simulink subsystem "RoboRio_Controls_sub"  (R2023b)
settings: Solver=VariableStepAuto  StartTime=0.0  StopTime=10.0  RelTol=1e-3
undefined symbols (not defined in the file): Odometry_IC_X, Odometry_IC_Y
libraries: simulink x4, Autonomous_lib x1, Disabled_lib x1, Teleop_lib x1, Test_lib x1
(part 1 of 2)
settings Model: Creator=USER  LastModifiedBy=ander

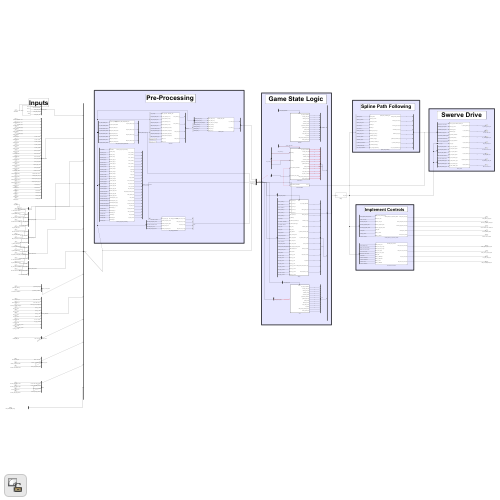
[thumbnail: Simulink's stored preview of the top-level diagram]
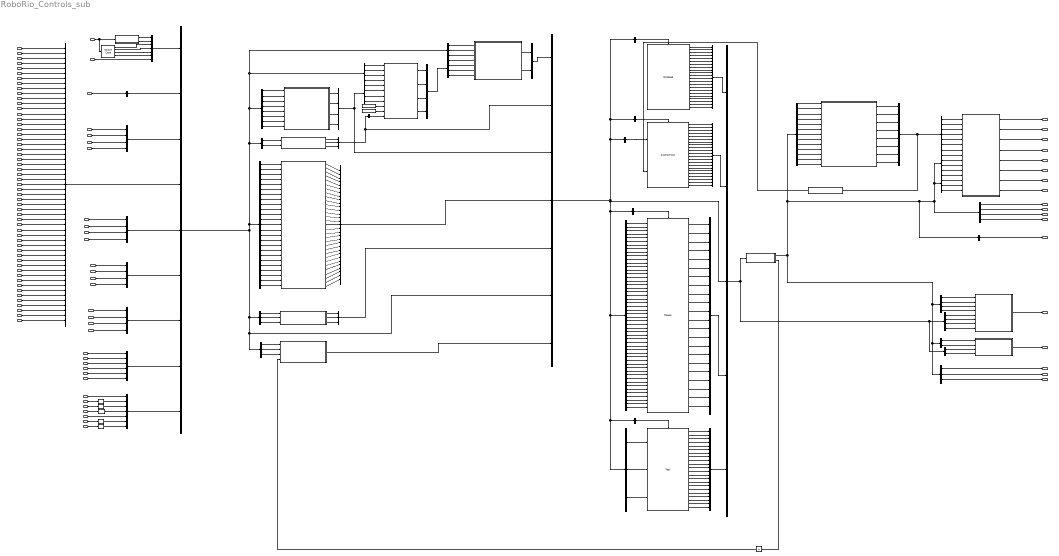
== system RoboRio_Controls_sub ==
  note: Game State Logic
  note: Swerve Drive
  note: Inputs
  note: Pre-Processing
  note: Spline Path
      | Following
  note: Reefscape
  GameState : Inport
  IsBlueAlliance : Inport  Port=2
  Joystick_Left_X : Inport  Port=3
  Joystick_Left_Y : Inport  Port=4
  Joystick_Left_Z : Inport  Port=5
  Joystick_Right_X : Inport  Port=6
  Joystick_Right_Y : Inport  Port=7
  Joystick_Right_Z : Inport  Port=8
  Joystick_Left_B1 : Inport  Port=9
  Joystick_Left_B2 : Inport  Port=10
  Joystick_Left_B3 : Inport  Port=11
  Joystick_Left_B4 : Inport  Port=12
  Joystick_Left_B5 : Inport  Port=13
  Joystick_Left_B6 : Inport  Port=14
  Joystick_Left_B7 : Inport  Port=15
  Joystick_Left_B8 : Inport  Port=16
  Joystick_Left_B9 : Inport  Port=17
  Joystick_Left_B10 : Inport  Port=18
  Joystick_Left_B11 : Inport  Port=19
  Joystick_Left_B12 : Inport  Port=20
  Joystick_Left_B13 : Inport  Port=21
  Joystick_Left_B14 : Inport  Port=22
  Joystick_Left_B15 : Inport  Port=23
  Joystick_Left_B16 : Inport  Port=24
  Joystick_Left_POV : Inport  Port=25
  Joystick_Right_B1 : Inport  Port=26
  Joystick_Right_B2 : Inport  Port=27
  Joystick_Right_B3 : Inport  Port=28
  Joystick_Right_B4 : Inport  Port=29
  Joystick_Right_B5 : Inport  Port=30
  Joystick_Right_B6 : Inport  Port=31
  Joystick_Right_B7 : Inport  Port=32
  Joystick_Right_B8 : Inport  Port=33
  Joystick_Right_B9 : Inport  Port=34
  Joystick_Right_B10 : Inport  Port=35
  Joystick_Right_B11 : Inport  Port=36
  Joystick_Right_B12 : Inport  Port=37
  Joystick_Right_B13 : Inport  Port=38
  Joystick_Right_B14 : Inport  Port=39
  Joystick_Right_B15 : Inport  Port=40
  Joystick_Right_B16 : Inport  Port=41
  Joystick_Right_POV : Inport  Port=42
  Gamepad_Stick_Left_X : Inport  Port=43
  Gamepad_Stick_Left_Y : Inport  Port=44
  Gamepad_Stick_Right_X : Inport  Port=45
  Gamepad_Stick_Right_Y : Inport  Port=46
  Gamepad_B1_A : Inport  Port=47
  Gamepad_B2_B : Inport  Port=48
  Gamepad_B3_X : Inport  Port=49
  Gamepad_B4_Y : Inport  Port=50
  Gamepad_LB : Inport  Port=51
  Gamepad_LT : Inport  Port=52
  Gamepad_RB : Inport  Port=53
  Gamepad_RT : Inport  Port=54
  Gamepad_Back : Inport  Port=55
  Gamepad_Start : Inport  Port=56
  Gamepad_POV : Inport  Port=57
  Gyro_Angle : Inport  Port=58
  FL_Drive_Motor_Speed : Inport  Port=59
  FR_Drive_Motor_Speed : Inport  Port=60
  BL_Drive_Motor_Speed : Inport  Port=61
  BR_Drive_Motor_Speed : Inport  Port=62
  FL_Drive_Motor_Rev : Inport  Port=63
  FR_Drive_Motor_Rev : Inport  Port=64
  BL_Drive_Motor_Rev : Inport  Port=65
  BR_Drive_Motor_Rev : Inport  Port=66
  FL_Steer_Module_Rev : Inport  Port=67
  FR_Steer_Module_Rev : Inport  Port=68
  BL_Steer_Module_Rev : Inport  Port=69
  BR_Steer_Module_Rev : Inport  Port=70
  FL_Steer_Module_Offset : Inport  Port=71
  FR_Steer_Module_Offset : Inport  Port=72
  BL_Steer_Module_Offset : Inport  Port=73
  BR_Steer_Module_Offset : Inport  Port=74
  Limelight_Est_Pose_X : Inport  Port=75
  Limelight_Est_Pose_Y : Inport  Port=76
  Num_Tags_Detected : Inport  Port=77
  Limelight_Tag_X : Inport  Port=78
  Limelight_Tag_Y : Inport  Port=79
  Limelight_Tag_Angle : Inport  Port=80
  Elevator_Motor_Rev : Inport  Port=81
  Elevator_Limit_Switch_Bottom : Inport  Port=82
  Elevator_Limit_Switch_Top : Inport  Port=83
  Coral_Arm_Angle_Measured_Raw : Inport  Port=84
  Coral_TOF_Distance : Inport  Port=85
  Coral_Limit_Switch : Inport  Port=86
  Algae_Limit_Switch : Inport  Port=87
  Add Constant : Bias  Bias=-180  SaturateOnIntegerOverflow=off
  Autonomous : Autonomous_lib/Autonomous  SystemSampleTime=-1  VariantActivationTime=update diagram  AllowFlexibleInterface=on  Latency=0  AutoFrameSizeCalculation=off
  Bus Creator : BusCreator  Inputs=7
  Bus Creator{1..2,4,12} (4 alike) : BusCreator  Inputs=22
  Bus Creator10 : BusCreator  Inputs=7
  Bus Creator11 : BusCreator  Inputs=9
  Bus Creator13 : BusCreator  Inputs=8
  Bus Creator{7..9,14..16} (6 alike) : BusCreator  Inputs=4
  Bus Creator17 : BusCreator  Inputs=7
  Bus Creator18 : BusCreator  Inputs=6
  Bus Creator19 : BusCreator  Inputs=2
  Bus Creator20 : BusCreator  Inputs=3
  Bus Creator21 : BusCreator  Inputs=3
  Bus Creator24 : BusCreator  Inputs=31
  Bus Creator3 : BusCreator  Inputs=5
  Bus Creator5 : BusCreator  Inputs=55
  Bus Creator6 : BusCreator  Inputs=1
  Bus Selector : BusSelector  OutputSignals=Steering_Abs_Cmd_SPF,Steering_Rel_Cmd_SPF,Translation_Speed_SPF,Translation_Angle_SPF,Is_Absolute_Translation_SPF,Is_Absolute_Steering_SPF,Gyro_Angle_SPF
  Bus Selector1 : BusSelector  OutputSignals=Odom_Position_X,Odom_Position_Y,Odom_Delta_X,Odom_Delta_Y
  Bus Selector10 : BusSelector  OutputSignals=Reefscape_Motors_Enable,Elevator_Height_Desired,Coral_Arm_Angle_Desired,Coral_Pickup_Lower_Wait_State
  Bus Selector11 : BusSelector  OutputSignals=Coral_Wheel_DutyCycle,Algae_Wheel_Outside_DutyCycle,Algae_Wheel_Inside_DutyCycle
  Bus Selector12 : BusSelector  OutputSignals=Reefscape_Motors_Enable,Coral_Arm_Angle_Desired
  Bus Selector13 : BusSelector  OutputSignals=Human_Inputs_Raw.Joystick_Left_X,Human_Inputs_Raw.Joystick_Left_Y,Human_Inputs_Raw.Joystick_Left_Z,Human_Inputs_Raw.Joystick_Right_X,Human_Inputs_Raw.Joystick_Right_Y,Human_Inputs_Raw.Joystick_Right_Z,Human_Inputs_Raw.Joystick_Left_B1,Human_Inputs_Raw.Joystick_Left_B2,Human_Inputs_Raw.Joystick_Left_B3,Human_Inputs_Raw.Joystick_Left_B4,Human_Inputs_Raw.Joystick_Left_B11,Human_Inputs_Raw.Joystick_Left_B12,Human_Inputs_Raw.Joystick_Left_B13,Human_Inputs_Raw.Joystick_Left_POV,Human_Inputs_Raw.Joystick_Right_B2,Human_Inputs_Raw.Joystick_Right_B3,Human_Inputs_Raw.Joystick_Right_B4,Human_Inputs_Raw.Joystick_Right_B5,Human_Inputs_Raw.Joystick_Right_B6,Human_Inputs_Raw.Joystick_Right_B7,Human_Inputs_Raw.Joystick_Right_B8,Human_Inputs_Raw.Joystick_Right_B9,Human_Inputs_Raw.Joystick_Right_B10,Human_Inputs_Raw.Joystick_Right_POV,Human_Inputs_Raw.Gamepad_POV
  Bus Selector14 : BusSelector  OutputSignals=PreProcessing.Inputs.Reefscape.Coral_Arm_Angle_Measured,PreProcessing.Elevator_Height_Measured
  Bus Selector15 : BusSelector  OutputSignals=PreProcessing.Gyro.Gyro_Angle_Offset_Total
  Bus Selector16 : BusSelector  OutputSignals=Human_Inputs_Processed.Button_Enable_Wheels,Human_Inputs_Processed.Button_Reset_Wheel_Offsets,Human_Inputs_Processed.Button_Disable_Wheels
  Bus Selector17 : BusSelector  OutputSignals=IMU_Sensor.Gyro_Angle_deg,Game_States.IsBlueAlliance
  Bus Selector18 : BusSelector  OutputSignals=Enable_Wheels,Reset_Wheel_Offsets,Disable_Wheels,Swerve_Motors_Disabled
  Bus Selector19 : BusSelector  OutputSignals=Gyro_Angle_Field_rad
  Bus Selector2 : BusSelector  OutputSignals=Inputs.Game_States.Game_State_Teleop
  Bus Selector20 : BusSelector  OutputSignals=Limelight_Estimates.Limelight_Tag_X,Limelight_Estimates.Limelight_Tag_Y,Limelight_Estimates.Limelight_Tag_Angle
  Bus Selector3 : BusSelector  OutputSignals=Limelight_Estimates.Limelight_Est_Pose_X,Limelight_Estimates.Limelight_Est_Pose_Y,Limelight_Estimates.Num_Tags_Detected
  Bus Selector4 : BusSelector  OutputSignals=Inputs.Game_States.Game_State_Auto
  Bus Selector40 : BusSelector  OutputSignals=Drive_Motor_Revs.FL_Drive_Motor_Rev,Drive_Motor_Revs.FR_Drive_Motor_Rev,Drive_Motor_Revs.BL_Drive_Motor_Rev,Drive_Motor_Revs.BR_Drive_Motor_Rev
  Bus Selector41 : BusSelector  OutputSignals=Human_Inputs_Processed.Drive_Joystick_X,Human_Inputs_Processed.Drive_Joystick_Y,Human_Inputs_Processed.Drive_Joystick_Z,Human_Inputs_Processed.Drive_Joystick_Z_Mode,Human_Inputs_Processed.Steer_Joystick_X,Human_Inputs_Processed.Steer_Joystick_Y,Human_Inputs_Processed.Steer_Joystick_Z,Human_Inputs_Processed.Is_Boosting,Human_Inputs_Processed.Face_Toward_Driver,Human_Inputs_Processed.Face_Right_Driver,Human_Inputs_Processed.Face_Left_Driver,Human_Inputs_Processed.Face_Away_Driver,Gyro.Gyro_Angle_rad,Inputs.Game_States.Prev_GameState,Inputs.Game_States.IsBlueAlliance,EKF.KF_Position_X,EKF.KF_Position_Y,Limelight_Tag_Corrected.Limelight_Tag_Corrected_X,Limelight_Tag_Corrected.Limelight_Tag_Corrected_Y,Limelight_Tag_Corrected.Limelight_Tag_Corrected_Angle,Human_Inputs_Processed.Align_Left,Human_Inputs_Processed.Align_Right,Human_Inputs_Processed.Align_Center,Human_Inputs_Processed.Coral_Station_Left,Human_Inputs_Processed.Coral_Station_Right,Human_Inputs_Processed.Processor,Human_Inputs_Processed.Cage_Left_Start,Human_Inputs_Processed.Cage_Middle_Start,Human_Inputs_Processed.Cage_Right_Start,Human_Inputs_Processed.Cage_Left_Finish,Human_Inputs_Processed.Cage_Middle_Finish,Human_Inputs_Processed.Cage_Right_Finish,Inputs.Human_Inputs_Raw.Gamepad_B1_A,Inputs.Human_Inputs_Raw.Gamepad_B2_B,Inputs.Human_Inputs_Raw.Gamepad_B3_X,Inputs.Human_Inputs_Raw.Gamepad_B4_Y,Inputs.Human_Inputs_Raw.Gamepad_Start,Inputs.Human_Inputs_Raw.Gamepad_Back,Inputs.Human_Inputs_Raw.Gamepad_RB,Inputs.Human_Inputs_Raw.Gamepad_LT,Inputs.Human_Inputs_Raw.Gamepad_RT,Human_Inputs_Processed.Gamepad_POV_Up,Human_Inputs_Processed.Gamepad_POV_Down,Human_Inputs_Processed.Gamepad_POV_Left,Human_Inputs_Processed.Gamepad_POV_Right,Inputs.Human_Inputs_Raw.Gamepad_Stick_Left_Y,Inputs.Human_Inputs_Raw.Gamepad_Stick_Right_Y,Elevator_Height_Measured,Inputs.Reefscape.Coral_Arm_Angle_Measured,Inputs.Reefscape.Coral_TOF_Distance,Inputs.Reefscape.Coral_Limit_Switch,Inputs.Reefscape.Algae_Limit_Switch
  Bus Selector5 : BusSelector  OutputSignals=Reefscape.Elevator_Motor_Rev,Reefscape.Elevator_Limit_Switch_Bottom,Reefscape.Elevator_Limit_Switch_Top
  Bus Selector50 : BusSelector  OutputSignals=PreProcessing.Inputs.Drive_Motor_Speeds.FL_Drive_Motor_Speed,PreProcessing.Inputs.Drive_Motor_Speeds.FR_Drive_Motor_Speed,PreProcessing.Inputs.Drive_Motor_Speeds.BL_Drive_Motor_Speed,PreProcessing.Inputs.Drive_Motor_Speeds.BR_Drive_Motor_Speed
  Bus Selector52 : BusSelector  OutputSignals=PreProcessing.Steer_Module_Angles.FL_Steer_Module_Angle,PreProcessing.Steer_Module_Angles.FR_Steer_Module_Angle,PreProcessing.Steer_Module_Angles.BL_Steer_Module_Angle,PreProcessing.Steer_Module_Angles.BR_Steer_Module_Angle
  Bus Selector57 : BusSelector  OutputSignals=Steer_Module_Revs.FL_Steer_Module_Rev,Steer_Module_Offsets.FL_Steer_Module_Offset,Steer_Module_Revs.FR_Steer_Module_Rev,Steer_Module_Offsets.FR_Steer_Module_Offset,Steer_Module_Revs.BL_Steer_Module_Rev,Steer_Module_Offsets.BL_Steer_Module_Offset,Steer_Module_Revs.BR_Steer_Module_Rev,Steer_Module_Offsets.BR_Steer_Module_Offset
  Bus Selector58 : BusSelector  OutputSignals=FL_Steer_Module_Angle,FR_Steer_Module_Angle,BL_Steer_Module_Angle,BR_Steer_Module_Angle
  Bus Selector59 : BusSelector  OutputSignals=Inputs.Game_States.IsBlueAlliance
  Bus Selector6 : BusSelector  OutputSignals=Inputs.Game_States.Game_State_Disabled
  Bus Selector7 : BusSelector  OutputSignals=PreProcessing.Elevator_Height_Measured,PreProcessing.Inputs.Reefscape.Elevator_Limit_Switch_Bottom,PreProcessing.Inputs.Reefscape.Elevator_Limit_Switch_Top,PreProcessing.Inputs.Reefscape.Coral_Arm_Angle_Measured
  Bus Selector8 : BusSelector  OutputSignals=Inputs.Game_States.Game_State_Test
  Bus Selector9 : BusSelector  OutputSignals=Spline_Enable,Spline_Ref_Poses,Spline_Num_Poses,PreProcessing.EKF.KF_Position_X,PreProcessing.EKF.KF_Position_Y,Steering_Abs_Cmd,Steering_Rel_Cmd,Translation_Speed,Translation_Angle,Is_Absolute_Translation,Is_Absolute_Steering,PreProcessing.Gyro.Gyro_Angle_Field_rad,PreProcessing.Gyro.Gyro_Angle_rad
  Compare To Zero{,1..3} (4 alike) : simulink/Logic and Bit Operations/Compare To Zero  relop=~=  OutDataTypeStr=boolean
  Constant : Constant  Value=Odometry_IC_X
  Constant1 : Constant  Value=Odometry_IC_Y
  Coral Arm Motor Control : Subsystem  ReferencedSubsystem=Coral_Arm_Motor_Control_sub
  Disabled : Disabled_lib/Disabled  SystemSampleTime=-1  VariantActivationTime=update diagram  AllowFlexibleInterface=on  Latency=0  AutoFrameSizeCalculation=off
  Elevator Motor Control : Subsystem  ReferencedSubsystem=Elevator_Motor_Control_sub
  Elevator_Height_Pre_Processing : Subsystem  ReferencedSubsystem=Elevator_Height_Pre_Processing_sub
  Gyro_Angles : Subsystem  ReferencedSubsystem=Gyro_Angles
  Human_Input_Pre_Processing : Subsystem  ReferencedSubsystem=Human_Input_Pre_Processing
  Internal Feedback : Subsystem
  Kalman_Filter : Subsystem  ReferencedSubsystem=Kalman_Filter_sub
  Limelight_Tag_Corrections : Subsystem  ReferencedSubsystem=Limelight_Tag_Corrections_sub
  Merge : Subsystem
  Odometry : Subsystem  ReferencedSubsystem=Odometry_sub
  Previous GameState : Subsystem
  Spline_Path_Following : Subsystem  ReferencedSubsystem=Spline_Path_Following_sub
  Steer_Module_Offset_Adjustments : Subsystem  ReferencedSubsystem=Steer_Module_Offset_Adjustments_sub
  Swerve_Drive : Subsystem  ReferencedSubsystem=Swerve_Drive_sub
  Switch Case : SwitchCase  CaseConditions={0,1,2}
  Teleop : Teleop_lib/Teleop  SystemSampleTime=-1  VariantActivationTime=update diagram  AllowFlexibleInterface=on  Latency=0  AutoFrameSizeCalculation=off
  Test : Test_lib/Test  SystemSampleTime=-1  VariantActivationTime=update diagram  AllowFlexibleInterface=on  Latency=0  AutoFrameSizeCalculation=off
  Unit Delay : UnitDelay  SampleTime=-1  HasFrameUpgradeWarning=on
  FL_Steering_Motor_DC : Outport
  FL_Drive_Motor_DC : Outport  Port=2
  FR_Steering_Motor_DC : Outport  Port=3
  FR_Drive_Motor_DC : Outport  Port=4
  BL_Steering_Motor_DC : Outport  Port=5
  BL_Drive_Motor_DC : Outport  Port=6
  BR_Steering_Motor_DC : Outport  Port=7
  BR_Drive_Motor_DC : Outport  Port=8
  Enable_Wheels : Outport  Port=9
  Reset_Wheel_Offsets : Outport  Port=10
  Disable_Wheels : Outport  Port=11
  Swerve_Motors_Disabled : Outport  Port=12
  Gyro_Angle_Offset_Total : Outport  Port=13
  Elevator_DutyCycle : Outport  Port=14
  Coral_Arm_DutyCycle : Outport  Port=15
  Coral_Wheel_DutyCycle : Outport  Port=16
  Algae_Wheel_Outside_DutyCycle : Outport  Port=17
  Algae_Wheel_Inside_DutyCycle : Outport  Port=18
  wires:
  Bus Creator4/1 -> Bus Creator3/1  "Disabled"
  Bus Creator1/1 -> Bus Creator3/2  "Autonomous"
  Bus Creator2/1 -> Bus Creator3/4  "Teleop"
  Switch Case/1 -> Bus Creator/3  "Game_State_Disabled"
  Switch Case/2 -> Bus Creator/4  "Game_State_Auto"
  Switch Case/3 -> Bus Creator/5  "Game_State_Teleop"
  GameState/1 -> Previous GameState/1(GameState_in), Switch Case/1  "GameState"
  Bus Creator12/1 -> Bus Creator3/5  "Test"
  Switch Case/4 -> Bus Creator/6  "Game_State_Test"
  FL_Drive_Motor_Speed/1 -> Bus Creator7/1  "FL_Drive_Motor_Speed"
  FR_Drive_Motor_Speed/1 -> Bus Creator7/2  "FR_Drive_Motor_Speed"
  BL_Drive_Motor_Speed/1 -> Bus Creator7/3  "BL_Drive_Motor_Speed"
  BR_Drive_Motor_Speed/1 -> Bus Creator7/4  "BR_Drive_Motor_Speed"
  FL_Steer_Module_Rev/1 -> Bus Creator8/1  "FL_Steer_Module_Rev"
  BL_Steer_Module_Rev/1 -> Bus Creator8/3  "BL_Steer_Module_Rev"
  BR_Steer_Module_Rev/1 -> Bus Creator8/4  "BR_Steer_Module_Rev"
  FR_Steer_Module_Rev/1 -> Bus Creator8/2  "FR_Steer_Module_Rev"
  Bus Creator7/1 -> Bus Creator11/3  "Drive_Motor_Speeds"
  Bus Creator8/1 -> Bus Creator11/6  "Steer_Module_Revs"
  FL_Steer_Module_Offset/1 -> Bus Creator9/1  "FL_Steer_Module_Offset"
  FR_Steer_Module_Offset/1 -> Bus Creator9/2  "FR_Steer_Module_Offset"
  BL_Steer_Module_Offset/1 -> Bus Creator9/3  "BL_Steer_Module_Offset"
  BR_Steer_Module_Offset/1 -> Bus Creator9/4  "BR_Steer_Module_Offset"
  Bus Creator9/1 -> Bus Creator11/7  "Steer_Module_Offsets"
  Bus Creator/1 -> Bus Creator11/1  "Game_States"
  Bus Selector2/1 -> Teleop/Action  "<Game_State_Teleop>"
  Bus Selector4/1 -> Autonomous/Action  "<Game_State_Auto>"
  Bus Selector6/1 -> Disabled/Action  "<Game_State_Disabled>"
  Bus Selector8/1 -> Test/Action  "<Game_State_Test>"
  Bus Selector50/4 -> Swerve_Drive/11  "<BR_Drive_Motor_Speed>"
  Bus Selector50/3 -> Swerve_Drive/10  "<BL_Drive_Motor_Speed>"
  Bus Selector50/2 -> Swerve_Drive/9  "<FR_Drive_Motor_Speed>"
  Bus Selector50/1 -> Swerve_Drive/8  "<FL_Drive_Motor_Speed>"
  Swerve_Drive/1 -> FL_Steering_Motor_DC/1
  Swerve_Drive/2 -> FL_Drive_Motor_DC/1
  Swerve_Drive/3 -> FR_Steering_Motor_DC/1
  Swerve_Drive/4 -> FR_Drive_Motor_DC/1
  Swerve_Drive/5 -> BL_Steering_Motor_DC/1
  Swerve_Drive/6 -> BL_Drive_Motor_DC/1
  Swerve_Drive/7 -> BR_Steering_Motor_DC/1
  Swerve_Drive/8 -> BR_Drive_Motor_DC/1
  Joystick_Left_B1/1 -> Bus Creator5/7  "Joystick_Left_B1"
  Bus Creator14/1 -> Bus Creator11/5  "Drive_Motor_Revs"
  FL_Drive_Motor_Rev/1 -> Bus Creator14/1  "FL_Drive_Motor_Rev"
  FR_Drive_Motor_Rev/1 -> Bus Creator14/2  "FR_Drive_Motor_Rev"
  BL_Drive_Motor_Rev/1 -> Bus Creator14/3  "BL_Drive_Motor_Rev"
  BR_Drive_Motor_Rev/1 -> Bus Creator14/4  "BR_Drive_Motor_Rev"
  Bus Selector40/1 -> Odometry/1  "<FL_Drive_Motor_Rev>"
  Bus Selector40/2 -> Odometry/2  "<FR_Drive_Motor_Rev>"
  Bus Selector40/3 -> Odometry/3  "<BL_Drive_Motor_Rev>"
  Bus Selector40/4 -> Odometry/4  "<BR_Drive_Motor_Rev>"
  Constant1/1 -> Odometry/10
  Constant/1 -> Odometry/9
  Bus Selector57/1 -> Steer_Module_Offset_Adjustments/1  "<FL_Steer_Module_Rev>"
  Bus Selector57/2 -> Steer_Module_Offset_Adjustments/2  "<FL_Steer_Module_Offset>"
  Bus Selector57/3 -> Steer_Module_Offset_Adjustments/3  "<FR_Steer_Module_Rev>"
  Bus Selector57/4 -> Steer_Module_Offset_Adjustments/4  "<FR_Steer_Module_Offset>"
  Bus Selector57/5 -> Steer_Module_Offset_Adjustments/5  "<BL_Steer_Module_Rev>"
  Bus Selector57/6 -> Steer_Module_Offset_Adjustments/6  "<BL_Steer_Module_Offset>"
  Bus Selector57/7 -> Steer_Module_Offset_Adjustments/7  "<BR_Steer_Module_Rev>"
  Bus Selector57/8 -> Steer_Module_Offset_Adjustments/8  "<BR_Steer_Module_Offset>"
  Steer_Module_Offset_Adjustments/2 -> Bus Creator15/2
  Steer_Module_Offset_Adjustments/1 -> Bus Creator15/1
  Steer_Module_Offset_Adjustments/3 -> Bus Creator15/3
  Steer_Module_Offset_Adjustments/4 -> Bus Creator15/4
  Bus Creator15/1 -> Bus Selector58/1, Bus Creator17/3  "Steer_Module_Angles"
  Bus Selector58/1 -> Odometry/5  "<FL_Steer_Module_Angle>"
  Bus Selector58/2 -> Odometry/6  "<FR_Steer_Module_Angle>"
  Bus Selector58/3 -> Odometry/7  "<BL_Steer_Module_Angle>"
  Bus Selector58/4 -> Odometry/8  "<BR_Steer_Module_Angle>"
  Bus Creator16/1 -> Bus Selector1/1  "Odometry"
  Bus Creator11/1 -> Bus Selector20/1, Bus Selector5/1, Bus Creator17/6, Bus Selector17/1, Bus Selector57/1, Bus Selector3/1, Bus Selector40/1, Bus Selector13/1  "Inputs"
  Bus Selector52/1 -> Swerve_Drive/12  "<FL_Steer_Module_Angle>"
  Bus Selector52/2 -> Swerve_Drive/13  "<FR_Steer_Module_Angle>"
  Bus Selector52/3 -> Swerve_Drive/14  "<BL_Steer_Module_Angle>"
  Bus Selector52/4 -> Swerve_Drive/15  "<BR_Steer_Module_Angle>"
  Merge/1(Bus_Out) -> Bus Selector10/1, Bus Selector12/1, Bus Selector11/1, Bus Selector9/1, Bus Selector52/1, Bus Selector50/1, Bus Selector18/1, Bus Selector15/1
  Bus Creator3/1 -> Bus Selector7/1, Bus Selector14/1, Merge/1(Bus_In)
  Bus Selector9/1 -> Spline_Path_Following/1  "<Spline_Enable>"
  Bus Selector9/2 -> Spline_Path_Following/2  "<Spline_Ref_Poses>"
  Bus Selector9/3 -> Spline_Path_Following/3  "<Spline_Num_Poses>"
  Bus Selector9/6 -> Spline_Path_Following/6  "<Steering_Abs_Cmd>"
  Bus Selector9/7 -> Spline_Path_Following/7  "<Steering_Rel_Cmd>"
  Bus Selector9/8 -> Spline_Path_Following/8  "<Translation_Speed>"
  Bus Selector9/9 -> Spline_Path_Following/9  "<Translation_Angle>"
  Bus Selector9/10 -> Spline_Path_Following/10  "<Is_Absolute_Translation>"
  Bus Selector9/11 -> Spline_Path_Following/11  "<Is_Absolute_Steering>"
  Spline_Path_Following/2 -> Bus Creator13/2
  Spline_Path_Following/3 -> Bus Creator13/3
  Spline_Path_Following/4 -> Bus Creator13/4
  Spline_Path_Following/5 -> Bus Creator13/5
  Spline_Path_Following/6 -> Bus Creator13/6
  Spline_Path_Following/7 -> Bus Creator13/7
  Bus Creator13/1 -> Bus Selector/1, Internal Feedback/1(Bus_In)
  Bus Selector/5 -> Swerve_Drive/5  "<Is_Absolute_Translation_SPF>"
  Bus Selector/4 -> Swerve_Drive/4  "<Translation_Angle_SPF>"
  Bus Selector/6 -> Swerve_Drive/6  "<Is_Absolute_Steering_SPF>"
  Bus Selector/3 -> Swerve_Drive/3  "<Translation_Speed_SPF>"
  Bus Selector/2 -> Swerve_Drive/2  "<Steering_Rel_Cmd_SPF>"
  Bus Selector/1 -> Swerve_Drive/1  "<Steering_Abs_Cmd_SPF>"
  Spline_Path_Following/1 -> Bus Creator13/1
  Limelight_Est_Pose_X/1 -> Bus Creator18/1  "Limelight_Est_Pose_X"
  Limelight_Est_Pose_Y/1 -> Bus Creator18/2  "Limelight_Est_Pose_Y"
  Num_Tags_Detected/1 -> Bus Creator18/3  "Num_Tags_Detected"
  Bus Selector1/3 -> Kalman_Filter/6  "<Odom_Delta_X>"
  Bus Selector1/4 -> Kalman_Filter/7  "<Odom_Delta_Y>"
  Bus Selector3/3 -> Kalman_Filter/3  "<Num_Tags_Detected>"
  Bus Selector3/2 -> Kalman_Filter/2  "<Limelight_Est_Pose_Y>"
  Bus Selector3/1 -> Kalman_Filter/1  "<Limelight_Est_Pose_X>"
  Kalman_Filter/1 -> Bus Creator19/1
  Kalman_Filter/2 -> Bus Creator19/2
  Bus Selector9/4 -> Spline_Path_Following/4  "<KF_Position_X>"
  Bus Selector9/5 -> Spline_Path_Following/5  "<KF_Position_Y>"
  Bus Creator19/1 -> Bus Creator17/1  "EKF"
  Odometry/1 -> Bus Creator16/1
  Odometry/2 -> Bus Creator16/2
  Odometry/3 -> Bus Creator16/3
  Odometry/4 -> Bus Creator16/4
  Bus Selector1/2 -> Kalman_Filter/5  "<Odom_Position_Y>"
  Bus Selector1/1 -> Kalman_Filter/4  "<Odom_Position_X>"
  Joystick_Left_B4/1 -> Bus Creator5/10  "Joystick_Left_B4"
  Joystick_Left_B3/1 -> Bus Creator5/9  "Joystick_Left_B3"
  Joystick_Left_B2/1 -> Bus Creator5/8  "Joystick_Left_B2"
  Bus Selector13/4 -> Human_Input_Pre_Processing/4  "<Joystick_Right_X>"
  Bus Selector13/5 -> Human_Input_Pre_Processing/5  "<Joystick_Right_Y>"
  Bus Selector13/1 -> Human_Input_Pre_Processing/1  "<Joystick_Left_X>"
  Bus Selector13/3 -> Human_Input_Pre_Processing/3  "<Joystick_Left_Z>"
  Bus Selector13/2 -> Human_Input_Pre_Processing/2  "<Joystick_Left_Y>"
  Bus Selector13/6 -> Human_Input_Pre_Processing/6  "<Joystick_Right_Z>"
  Bus Selector13/7 -> Human_Input_Pre_Processing/7  "<Joystick_Left_B1>"
  Bus Selector13/8 -> Human_Input_Pre_Processing/8  "<Joystick_Left_B2>"
  Bus Selector13/9 -> Human_Input_Pre_Processing/9  "<Joystick_Left_B3>"
  Bus Selector13/10 -> Human_Input_Pre_Processing/10  "<Joystick_Left_B4>"
  Joystick_Left_Y/1 -> Bus Creator5/2  "Joystick_Left_Y"
  Joystick_Left_X/1 -> Bus Creator5/1  "Joystick_Left_X"
  Joystick_Left_Z/1 -> Bus Creator5/3  "Joystick_Left_Z"
  Joystick_Right_X/1 -> Bus Creator5/4  "Joystick_Right_X"
  Joystick_Right_Y/1 -> Bus Creator5/5  "Joystick_Right_Y"
  Joystick_Right_Z/1 -> Bus Creator5/6  "Joystick_Right_Z"
  Bus Creator24/1 -> Bus Creator17/4  "Human_Inputs_Processed"
  Bus Creator17/1 -> Bus Selector59/1, Bus Selector4/1, Bus Selector6/1, Bus Creator3/3, Bus Selector2/1, Bus Selector41/1, Bus Selector8/1, Bus Selector16/1  "PreProcessing"
  Bus Creator18/1 -> Bus Creator11/8  "Limelight_Estimates"
  Internal Feedback/1(Robot_Reached_Destination) -> Autonomous/2
  Limelight_Tag_X/1 -> Bus Creator18/4  "Limelight_Tag_X"
  Limelight_Tag_Y/1 -> Bus Creator18/5  "Limelight_Tag_Y"
  Limelight_Tag_Angle/1 -> Bus Creator18/6  "Limelight_Tag_Angle"
  Previous GameState/1(GameState) -> Bus Creator/1
  Previous GameState/2(Prev_GameState) -> Bus Creator/2
  Gyro_Angle/1 -> Bus Creator6/1  "Gyro_Angle_deg"
  IsBlueAlliance/1 -> Bus Creator/7  "IsBlueAlliance"
  Bus Selector17/2 -> Gyro_Angles/2  "<IsBlueAlliance>"
  Bus Selector17/1 -> Gyro_Angles/1  "<Gyro_Angle_deg>"
  Gyro_Angles/1 -> Bus Creator20/1
  Gyro_Angles/2 -> Bus Creator20/2
  Bus Creator20/1 -> Bus Creator17/2, Bus Selector19/1  "Gyro"
  Bus Selector19/1 -> Odometry/11  "<Gyro_Angle_Field_rad>"
  Bus Selector9/12 -> Spline_Path_Following/12  "<Gyro_Angle_Field_rad>"
  Bus Selector9/13 -> Spline_Path_Following/13  "<Gyro_Angle_rad>"
  Spline_Path_Following/8 -> Bus Creator13/8
  Bus Selector/7 -> Swerve_Drive/7  "<Gyro_Angle_SPF>"
  Bus Selector59/1 -> Autonomous/1  "<IsBlueAlliance>"
  Disabled/1 -> Bus Creator4/1
  Disabled/2 -> Bus Creator4/2
  Disabled/3 -> Bus Creator4/3
  Disabled/4 -> Bus Creator4/4
  Disabled/5 -> Bus Creator4/5
  Disabled/6 -> Bus Creator4/6
  Disabled/7 -> Bus Creator4/7
  Disabled/8 -> Bus Creator4/8
  Disabled/9 -> Bus Creator4/9
  Autonomous/1 -> Bus Creator1/1
  Autonomous/2 -> Bus Creator1/2
  Autonomous/3 -> Bus Creator1/3
  Autonomous/4 -> Bus Creator1/4
  Autonomous/5 -> Bus Creator1/5
  Autonomous/6 -> Bus Creator1/6
  Autonomous/7 -> Bus Creator1/7
  Autonomous/8 -> Bus Creator1/8
  Autonomous/9 -> Bus Creator1/9
  Autonomous/10 -> Bus Creator1/10
  Teleop/1 -> Bus Creator2/1
  Teleop/2 -> Bus Creator2/2
  Teleop/3 -> Bus Creator2/3
  Teleop/4 -> Bus Creator2/4
  Teleop/5 -> Bus Creator2/5
  Teleop/6 -> Bus Creator2/6
  Teleop/7 -> Bus Creator2/7
  Teleop/8 -> Bus Creator2/8
  Teleop/9 -> Bus Creator2/9
  Teleop/10 -> Bus Creator2/10
  Teleop/11 -> Bus Creator2/11
  Teleop/12 -> Bus Creator2/12
  Teleop/13 -> Bus Creator2/13
  Test/1 -> Bus Creator12/1
  Test/2 -> Bus Creator12/2
  Test/3 -> Bus Creator12/3
  Test/4 -> Bus Creator12/4
  Test/5 -> Bus Creator12/5
  Test/6 -> Bus Creator12/6
  Test/7 -> Bus Creator12/7
  Test/8 -> Bus Creator12/8
  Test/9 -> Bus Creator12/9
  Test/10 -> Bus Creator12/10
  Teleop/14 -> Bus Creator2/14
  Bus Selector18/2 -> Reset_Wheel_Offsets/1  "<Reset_Wheel_Offsets>"
  Bus Selector18/3 -> Disable_Wheels/1  "<Disable_Wheels>"
  Bus Selector18/4 -> Swerve_Motors_Disabled/1  "<Swerve_Motors_Disabled>"
  Bus Selector18/1 -> Enable_Wheels/1  "<Enable_Wheels>"
  Disabled/10 -> Bus Creator4/10
  Disabled/11 -> Bus Creator4/11
  Disabled/12 -> Bus Creator4/12
  Disabled/13 -> Bus Creator4/13
  Disabled/14 -> Bus Creator4/14
  Autonomous/11 -> Bus Creator1/11
  Autonomous/12 -> Bus Creator1/12
  Autonomous/13 -> Bus Creator1/13
  Autonomous/14 -> Bus Creator1/14
  Test/11 -> Bus Creator12/11
  Test/12 -> Bus Creator12/12
  Test/13 -> Bus Creator12/13
  Test/14 -> Bus Creator12/14
  Bus Selector16/1 -> Test/1  "<Button_Enable_Wheels>"
  Bus Selector16/2 -> Test/2  "<Button_Reset_Wheel_Offsets>"
  Bus Selector16/3 -> Test/3  "<Button_Disable_Wheels>"
  Joystick_Left_B5/1 -> Bus Creator5/11  "Joystick_Left_B5"
  Joystick_Left_B6/1 -> Bus Creator5/12  "Joystick_Left_B6"
  Joystick_Left_B7/1 -> Bus Creator5/13  "Joystick_Left_B7"
  Joystick_Left_B8/1 -> Bus Creator5/14  "Joystick_Left_B8"
  Joystick_Left_B9/1 -> Bus Creator5/15  "Joystick_Left_B9"
  Joystick_Left_B10/1 -> Bus Creator5/16  "Joystick_Left_B10"
  Joystick_Left_B11/1 -> Bus Creator5/17  "Joystick_Left_B11"
  Joystick_Left_B12/1 -> Bus Creator5/18  "Joystick_Left_B12"
  Joystick_Left_B13/1 -> Bus Creator5/19  "Joystick_Left_B13"
  Joystick_Left_B14/1 -> Bus Creator5/20  "Joystick_Left_B14"
  Joystick_Left_B15/1 -> Bus Creator5/21  "Joystick_Left_B15"
  Joystick_Left_B16/1 -> Bus Creator5/22  "Joystick_Left_B16"
  Joystick_Left_POV/1 -> Bus Creator5/23  "Joystick_Left_POV"
  Joystick_Right_B1/1 -> Bus Creator5/24  "Joystick_Right_B1"
  Joystick_Right_B2/1 -> Bus Creator5/25  "Joystick_Right_B2"
  Joystick_Right_B3/1 -> Bus Creator5/26  "Joystick_Right_B3"
  Joystick_Right_B4/1 -> Bus Creator5/27  "Joystick_Right_B4"
  Joystick_Right_B5/1 -> Bus Creator5/28  "Joystick_Right_B5"
  Joystick_Right_B6/1 -> Bus Creator5/29  "Joystick_Right_B6"
  Joystick_Right_B7/1 -> Bus Creator5/30  "Joystick_Right_B7"
  Joystick_Right_B8/1 -> Bus Creator5/31  "Joystick_Right_B8"
  Joystick_Right_B9/1 -> Bus Creator5/32  "Joystick_Right_B9"
  Joystick_Right_B10/1 -> Bus Creator5/33  "Joystick_Right_B10"
  Joystick_Right_B11/1 -> Bus Creator5/34  "Joystick_Right_B11"
  Joystick_Right_B12/1 -> Bus Creator5/35  "Joystick_Right_B12"
  Joystick_Right_B13/1 -> Bus Creator5/36  "Joystick_Right_B13"
  Joystick_Right_B14/1 -> Bus Creator5/37  "Joystick_Right_B14"
  Joystick_Right_B15/1 -> Bus Creator5/38  "Joystick_Right_B15"
  Joystick_Right_B16/1 -> Bus Creator5/39  "Joystick_Right_B16"
  Joystick_Right_POV/1 -> Bus Creator5/40  "Joystick_Right_POV"
  Gamepad_Stick_Left_X/1 -> Bus Creator5/41  "Gamepad_Stick_Left_X"
  Gamepad_Stick_Left_Y/1 -> Bus Creator5/42  "Gamepad_Stick_Left_Y"
  Gamepad_Stick_Right_X/1 -> Bus Creator5/43  "Gamepad_Stick_Right_X"
  Gamepad_Stick_Right_Y/1 -> Bus Creator5/44  "Gamepad_Stick_Right_Y"
  Gamepad_B1_A/1 -> Bus Creator5/45  "Gamepad_B1_A"
  Gamepad_B2_B/1 -> Bus Creator5/46  "Gamepad_B2_B"
  Gamepad_B3_X/1 -> Bus Creator5/47  "Gamepad_B3_X"
  Gamepad_B4_Y/1 -> Bus Creator5/48  "Gamepad_B4_Y"
  Gamepad_LB/1 -> Bus Creator5/49  "Gamepad_LB"
  Gamepad_LT/1 -> Bus Creator5/50  "Gamepad_LT"
  Gamepad_RB/1 -> Bus Creator5/51  "Gamepad_RB"
  Gamepad_RT/1 -> Bus Creator5/52  "Gamepad_RT"
  Gamepad_Back/1 -> Bus Creator5/53  "Gamepad_Back"
  Gamepad_Start/1 -> Bus Creator5/54  "Gamepad_Start"
  Bus Creator6/1 -> Bus Creator11/2  "IMU_Sensor"
  Bus Creator5/1 -> Bus Creator11/4  "Human_Inputs_Raw"
  Elevator_Motor_Rev/1 -> Bus Creator10/1  "Elevator_Motor_Rev"
  Elevator_Limit_Switch_Bottom/1 -> Compare To Zero/1
  Elevator_Limit_Switch_Top/1 -> Compare To Zero1/1
  Bus Creator10/1 -> Bus Creator11/9  "Reefscape"
  Bus Selector7/1 -> Elevator Motor Control/5  "<Elevator_Height_Measured>"
  Bus Selector7/2 -> Elevator Motor Control/6  "<Elevator_Limit_Switch_Bottom>"
  Bus Selector7/3 -> Elevator Motor Control/7  "<Elevator_Limit_Switch_Top>"
  Elevator Motor Control/1 -> Elevator_DutyCycle/1
  Bus Selector5/1 -> Elevator_Height_Pre_Processing/1  "<Elevator_Motor_Rev>"
  Elevator_Height_Pre_Processing/1 -> Bus Creator17/7
  Compare To Zero/1 -> Bus Creator10/2  "Elevator_Limit_Switch_Bottom"
  Compare To Zero1/1 -> Bus Creator10/3  "Elevator_Limit_Switch_Top"
  Disabled/15 -> Bus Creator4/15
  Disabled/16 -> Bus Creator4/16
  Autonomous/15 -> Bus Creator1/15
  Autonomous/16 -> Bus Creator1/16
  Teleop/15 -> Bus Creator2/15
  Teleop/16 -> Bus Creator2/16
  Test/15 -> Bus Creator12/15
  Test/16 -> Bus Creator12/16
  Bus Selector10/2 -> Elevator Motor Control/2  "<Elevator_Height_Desired>"
  Bus Selector10/1 -> Elevator Motor Control/1  "<Reefscape_Motors_Enable>"
  Bus Selector5/2 -> Elevator_Height_Pre_Processing/2  "<Elevator_Limit_Switch_Bottom>"
  Gamepad_POV/1 -> Bus Creator5/55  "Gamepad_POV"
  Coral_TOF_Distance/1 -> Bus Creator10/5  "Coral_TOF_Distance"
  Coral_Limit_Switch/1 -> Compare To Zero2/1
  Coral_Arm_Angle_Measured_Raw/1 -> Add Constant/1
  Compare To Zero2/1 -> Bus Creator10/6  "Coral_Limit_Switch"
  Teleop/17 -> Bus Creator2/17
  Teleop/18 -> Bus Creator2/18
  Disabled/17 -> Bus Creator4/17
  Disabled/18 -> Bus Creator4/18
  Autonomous/17 -> Bus Creator1/17
  Autonomous/18 -> Bus Creator1/18
  Test/17 -> Bus Creator12/17
  Test/18 -> Bus Creator12/18
  Bus Selector12/1 -> Coral Arm Motor Control/1  "<Reefscape_Motors_Enable>"
  Bus Selector12/2 -> Coral Arm Motor Control/2  "<Coral_Arm_Angle_Desired>"
  Coral Arm Motor Control/1 -> Coral_Arm_DutyCycle/1
  Bus Selector14/1 -> Coral Arm Motor Control/3  "<Coral_Arm_Angle_Measured>"
  Bus Selector11/1 -> Coral_Wheel_DutyCycle/1  "<Coral_Wheel_DutyCycle>"
  Add Constant/1 -> Bus Creator10/4  "Coral_Arm_Angle_Measured"
  Algae_Limit_Switch/1 -> Compare To Zero3/1
  Compare To Zero3/1 -> Bus Creator10/7  "Algae_Limit_Switch"
  Teleop/19 -> Bus Creator2/19
  Teleop/20 -> Bus Creator2/20
  Disabled/19 -> Bus Creator4/19
  Disabled/20 -> Bus Creator4/20
  Autonomous/19 -> Bus Creator1/19
  Autonomous/20 -> Bus Creator1/20
  Test/19 -> Bus Creator12/19
  Test/20 -> Bus Creator12/20
  Bus Selector11/2 -> Algae_Wheel_Outside_DutyCycle/1  "<Algae_Wheel_Outside_DutyCycle>"
  Bus Selector11/3 -> Algae_Wheel_Inside_DutyCycle/1  "<Algae_Wheel_Inside_DutyCycle>"
  Bus Selector7/4 -> Elevator Motor Control/8  "<Coral_Arm_Angle_Measured>"
  Bus Selector14/2 -> Coral Arm Motor Control/4  "<Elevator_Height_Measured>"
  Bus Selector10/3 -> Elevator Motor Control/3  "<Coral_Arm_Angle_Desired>"
  Bus Selector5/3 -> Elevator_Height_Pre_Processing/3  "<Elevator_Limit_Switch_Top>"
  Disabled/21 -> Bus Creator4/21
  Autonomous/21 -> Bus Creator1/21
  Teleop/21 -> Bus Creator2/21
  Test/21 -> Bus Creator12/21
  Merge/2(Elevator_LowerPickup_Reset) -> Unit Delay/1
  Unit Delay/1 -> Elevator_Height_Pre_Processing/4
  Disabled/22 -> Bus Creator4/22
  Autonomous/22 -> Bus Creator1/22
  Teleop/22 -> Bus Creator2/22
  Test/22 -> Bus Creator12/22
  Bus Selector10/4 -> Elevator Motor Control/4  "<Coral_Pickup_Lower_Wait_State>"
  Gyro_Angles/3 -> Bus Creator20/3
  Bus Selector15/1 -> Gyro_Angle_Offset_Total/1  "<Gyro_Angle_Offset_Total>"
  Bus Selector20/1 -> Limelight_Tag_Corrections/1  "<Limelight_Tag_X>"
  Bus Selector20/2 -> Limelight_Tag_Corrections/2  "<Limelight_Tag_Y>"
  Bus Selector20/3 -> Limelight_Tag_Corrections/3  "<Limelight_Tag_Angle>"
  Limelight_Tag_Corrections/1 -> Bus Creator21/1
  Limelight_Tag_Corrections/2 -> Bus Creator21/2
  Limelight_Tag_Corrections/3 -> Bus Creator21/3
  Bus Creator21/1 -> Bus Creator17/5  "Limelight_Tag_Corrected"
  Human_Input_Pre_Processing/1 -> Bus Creator24/1
  Human_Input_Pre_Processing/2 -> Bus Creator24/2
  Human_Input_Pre_Processing/3 -> Bus Creator24/3
  Human_Input_Pre_Processing/4 -> Bus Creator24/4
  Human_Input_Pre_Processing/5 -> Bus Creator24/5
  Human_Input_Pre_Processing/6 -> Bus Creator24/6
  Human_Input_Pre_Processing/7 -> Bus Creator24/7
  Human_Input_Pre_Processing/8 -> Bus Creator24/8
  Human_Input_Pre_Processing/9 -> Bus Creator24/9
  Human_Input_Pre_Processing/10 -> Bus Creator24/10
  Human_Input_Pre_Processing/11 -> Bus Creator24/11
  Human_Input_Pre_Processing/12 -> Bus Creator24/12
  Human_Input_Pre_Processing/13 -> Bus Creator24/13
  Human_Input_Pre_Processing/14 -> Bus Creator24/14
  Human_Input_Pre_Processing/15 -> Bus Creator24/15
  Human_Input_Pre_Processing/16 -> Bus Creator24/16
  Human_Input_Pre_Processing/17 -> Bus Creator24/17
  Human_Input_Pre_Processing/18 -> Bus Creator24/18
  Human_Input_Pre_Processing/19 -> Bus Creator24/19
  Human_Input_Pre_Processing/20 -> Bus Creator24/20
  Human_Input_Pre_Processing/21 -> Bus Creator24/21
  Human_Input_Pre_Processing/22 -> Bus Creator24/22
  Human_Input_Pre_Processing/23 -> Bus Creator24/23
  Human_Input_Pre_Processing/24 -> Bus Creator24/24
  Human_Input_Pre_Processing/25 -> Bus Creator24/25
  Bus Selector41/1 -> Teleop/1  "<Drive_Joystick_X>"
  Bus Selector13/11 -> Human_Input_Pre_Processing/11  "<Joystick_Left_B11>"
  Bus Selector13/12 -> Human_Input_Pre_Processing/12  "<Joystick_Left_B12>"
  Bus Selector13/13 -> Human_Input_Pre_Processing/13  "<Joystick_Left_B13>"
  Bus Selector13/14 -> Human_Input_Pre_Processing/14  "<Joystick_Left_POV>"
  Bus Selector13/15 -> Human_Input_Pre_Processing/15  "<Joystick_Right_B2>"
  Bus Selector13/16 -> Human_Input_Pre_Processing/16  "<Joystick_Right_B3>"
  Bus Selector13/17 -> Human_Input_Pre_Processing/17  "<Joystick_Right_B4>"
  Bus Selector13/18 -> Human_Input_Pre_Processing/18  "<Joystick_Right_B5>"
  Bus Selector13/19 -> Human_Input_Pre_Processing/19  "<Joystick_Right_B6>"
  Bus Selector13/20 -> Human_Input_Pre_Processing/20  "<Joystick_Right_B7>"
  Bus Selector13/21 -> Human_Input_Pre_Processing/21  "<Joystick_Right_B8>"
  Bus Selector13/22 -> Human_Input_Pre_Processing/22  "<Joystick_Right_B9>"
  Bus Selector13/23 -> Human_Input_Pre_Processing/23  "<Joystick_Right_B10>"
  Bus Selector13/24 -> Human_Input_Pre_Processing/24  "<Joystick_Right_POV>"
  Bus Selector13/25 -> Human_Input_Pre_Processing/25  "<Gamepad_POV>"
  Human_Input_Pre_Processing/26 -> Bus Creator24/26
  Human_Input_Pre_Processing/27 -> Bus Creator24/27
  Human_Input_Pre_Processing/28 -> Bus Creator24/28
  Human_Input_Pre_Processing/29 -> Bus Creator24/29
  Human_Input_Pre_Processing/30 -> Bus Creator24/30
  Human_Input_Pre_Processing/31 -> Bus Creator24/31
  Bus Selector41/2 -> Teleop/2  "<Drive_Joystick_Y>"
  Bus Selector41/3 -> Teleop/3  "<Drive_Joystick_Z>"
  Bus Selector41/4 -> Teleop/4  "<Drive_Joystick_Z_Mode>"
  Bus Selector41/5 -> Teleop/5  "<Steer_Joystick_X>"
  Bus Selector41/6 -> Teleop/6  "<Steer_Joystick_Y>"
  Bus Selector41/7 -> Teleop/7  "<Steer_Joystick_Z>"
  Bus Selector41/8 -> Teleop/8  "<Is_Boosting>"
  Bus Selector41/9 -> Teleop/9  "<Face_Toward_Driver>"
  Bus Selector41/10 -> Teleop/10  "<Face_Right_Driver>"
  Bus Selector41/11 -> Teleop/11  "<Face_Left_Driver>"
  Bus Selector41/12 -> Teleop/12  "<Face_Away_Driver>"
  Bus Selector41/13 -> Teleop/13  "<Gyro_Angle_rad>"
  Bus Selector41/14 -> Teleop/14  "<Prev_GameState>"
  Bus Selector41/15 -> Teleop/15  "<IsBlueAlliance>"
  Bus Selector41/16 -> Teleop/16  "<KF_Position_X>"
  Bus Selector41/17 -> Teleop/17  "<KF_Position_Y>"
  Bus Selector41/18 -> Teleop/18  "<Limelight_Tag_Corrected_X>"
  Bus Selector41/19 -> Teleop/19  "<Limelight_Tag_Corrected_Y>"
  Bus Selector41/20 -> Teleop/20  "<Limelight_Tag_Corrected_Angle>"
  Bus Selector41/21 -> Teleop/21  "<Align_Left>"
  Bus Selector41/22 -> Teleop/22  "<Align_Right>"
  Bus Selector41/23 -> Teleop/23  "<Align_Center>"
  Bus Selector41/24 -> Teleop/24  "<Coral_Station_Left>"
  Bus Selector41/25 -> Teleop/25  "<Coral_Station_Right>"
  Bus Selector41/26 -> Teleop/26  "<Processor>"
  Bus Selector41/27 -> Teleop/27  "<Cage_Left_Start>"
  Bus Selector41/28 -> Teleop/28  "<Cage_Middle_Start>"
  Bus Selector41/29 -> Teleop/29  "<Cage_Right_Start>"
  Bus Selector41/30 -> Teleop/30  "<Cage_Left_Finish>"
  Bus Selector41/31 -> Teleop/31  "<Cage_Middle_Finish>"
  Bus Selector41/32 -> Teleop/32  "<Cage_Right_Finish>"
  Bus Selector41/33 -> Teleop/33  "<Gamepad_B1_A>"
  Bus Selector41/34 -> Teleop/34  "<Gamepad_B2_B>"
  Bus Selector41/35 -> Teleop/35  "<Gamepad_B3_X>"
  Bus Selector41/36 -> Teleop/36  "<Gamepad_B4_Y>"
  Bus Selector41/37 -> Teleop/37  "<Gamepad_Start>"
  Bus Selector41/38 -> Teleop/38  "<Gamepad_Back>"
  Bus Selector41/39 -> Teleop/39  "<Gamepad_RB>"
  Bus Selector41/40 -> Teleop/40  "<Gamepad_LT>"
  Bus Selector41/41 -> Teleop/41  "<Gamepad_RT>"
  Bus Selector41/42 -> Teleop/42  "<Gamepad_POV_Up>"
  Bus Selector41/43 -> Teleop/43  "<Gamepad_POV_Down>"
  Bus Selector41/44 -> Teleop/44  "<Gamepad_POV_Left>"
  Bus Selector41/45 -> Teleop/45  "<Gamepad_POV_Right>"
  Bus Selector41/46 -> Teleop/46  "<Gamepad_Stick_Left_Y>"
  Bus Selector41/47 -> Teleop/47  "<Gamepad_Stick_Right_Y>"
  Bus Selector41/48 -> Teleop/48  "<Elevator_Height_Measured>"
  Bus Selector41/49 -> Teleop/49  "<Coral_Arm_Angle_Measured>"
  Bus Selector41/50 -> Teleop/50  "<Coral_TOF_Distance>"
  Bus Selector41/51 -> Teleop/51  "<Coral_Limit_Switch>"
  Bus Selector41/52 -> Teleop/52  "<Algae_Limit_Switch>"

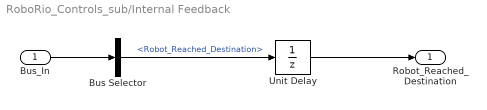
== system RoboRio_Controls_sub/Internal Feedback ==
  Bus_In : Inport
  Bus Selector : BusSelector  OutputSignals=Robot_Reached_Destination
  Unit Delay : UnitDelay  SampleTime=-1  HasFrameUpgradeWarning=on
  Robot_Reached_Destination : Outport
  wires:
  Unit Delay/1 -> Robot_Reached_Destination/1
  Bus Selector/1 -> Unit Delay/1  "<Robot_Reached_Destination>"
  Bus_In/1 -> Bus Selector/1
